simulink model "ur5bh_JustFollow"  (R2021b)
settings: Solver=ode23  StartTime=0.0  StopTime=13  FixedStep=1e-4  MaxStep=1e-3  RelTol=1e-2  AbsTol=1e-2
values from neighbouring files (symbols this model uses):
  Act_Hand = zeros(Phase_Num,1)    [Event2Action.m]
  Act_Lift = zeros(Phase_Num,1)    [Event2Action.m]
  Act_Planner = zeros(Phase_Num,1)    [Event2Action.m]
  Act_Time = zeros(Phase_Num,1)    [Event2Action.m]
  Act_XYZ = zeros(Phase_Num,3)    [Event2Action.m]
  Act_YPR = zeros(Phase_Num,3)    [Event2Action.m]
  maxIter = 200    [Fri_Lancher.m]    (also in ur5bhLancher.m)
undefined symbols (not defined in the file or in its folder): X, Y, Z
libraries: sm_lib x186, nesl_utility x38, robotmaniplib x2, simulink x1
(part 1 of 5)
settings Model: Creator=jobs  LastModifiedBy=jobs

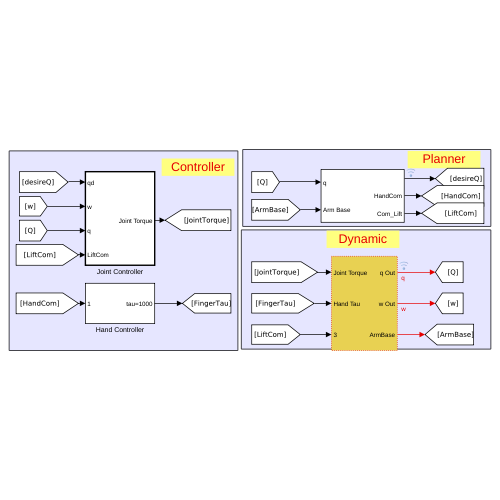
[thumbnail: Simulink's stored preview of the top-level diagram]
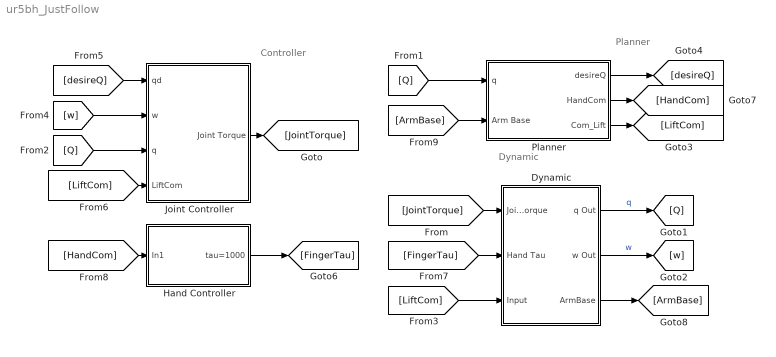
== system ur5bh_JustFollow ==
  note: Dynamic
  note: Planner
  note: Controller
  Dynamic : Subsystem
      settings: MinAlgLoopOccurrences=on
  Hand Controller : Subsystem
  Joint Controller : Subsystem  TreatAsAtomicUnit=on  SystemSampleTime=1e-3
  Planner : Subsystem
  wires:
  Joint Controller/1(Joint Torque) -> [JointTorque]
  [JointTorque] -> Dynamic/1(Joint Torque)
  [Q] -> Planner/1(q)
  [Q] -> Joint Controller/3(q)
  Dynamic/1(q Out) -> [Q]  "q"
  [w] -> Joint Controller/2(w)
  Dynamic/2(w Out) -> [w]  "w"
  Planner/1(desireQ) -> [desireQ]
  [desireQ] -> Joint Controller/1(qd)
  [FingerTau] -> Dynamic/2(Hand Tau)
  Planner/2(HandCom) -> [HandCom]
  [HandCom] -> Hand Controller/1(In1)
  Hand Controller/1(tau=1000) -> [FingerTau]
  Dynamic/3(ArmBase) -> [ArmBase]
  [ArmBase] -> Planner/2(Arm Base)
  [LiftCom] -> Dynamic/3(Input)
  Planner/3(Com_Lift) -> [LiftCom]
  [LiftCom] -> Joint Controller/4(LiftCom)

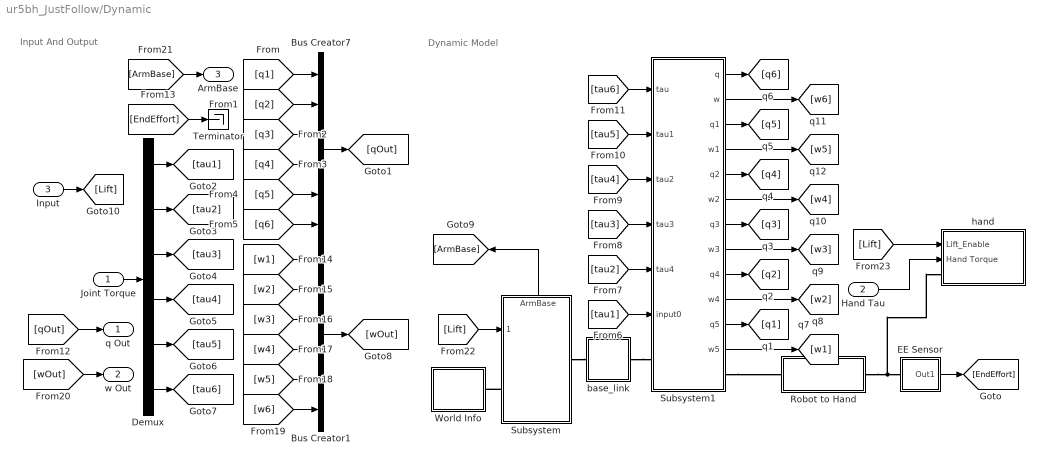
== system ur5bh_JustFollow/Dynamic ==
  note: Dynamic Model
  note: Input And Output
  Joint Torque : Inport
  Hand Tau : Inport  Port=2
  Input : Inport  Port=3
  Bus Creator1 : BusCreator  Inputs=6
  Bus Creator7 : BusCreator  Inputs=6
  Demux : Demux  Outputs=6
  EE Sensor : Subsystem
      settings: PortSchema="{\"entries\":[{\"content\":{\"sides\":[{\"content\":{\"connectorIds\":[\"Out1\"]},\"type\":\"ConnectorPlacement.EquallySpacedRectSide\",\"uuid\":\"1821bd9e-34df-46f7-8d9b-73402f01dbc0\"},{\"content\":{\"connectorIds\":[\"RConn1\"],\"side\":\"RIGHT\"},\"type\":\"ConnectorPlacement.EquallySpacedRectSide\",\"uuid\":\"cfe01d0d-0504-46d0-96c4-84d5e751aaf1\"},{\"content\":{\"connectorIds\":[],\"side\":\"TOP\"},\"type\":\"ConnectorPlacement.EquallySpacedRectSide\",\"uuid\":\"fb6ec0bf-6e00-4c48-b353-ee97f79f22fa\"},{\"content\":{\"connectorIds\":[],\"side\":\"BOTTOM\"},\"type\":\"ConnectorPlacement.EquallySpacedRectSide\",\"uuid\":\"6688a5de-4d5c-429f-9ca8-418d1bff595a\"}]},\"type\":\"ConnectorPlacement.EquallySpacedConnector\",\"uuid\":\"28678e19-8d3c-4397-9fe9-d3bc3a97349c\"}],\"packageUris\":[\"http://schema.mathworks.com/mf0/Connector/R2020b\"],\"version\":\"1.0\"}"
  Robot to Hand : Subsystem
  Subsystem : Subsystem
      settings: PortSchema="{\"entries\":[{\"content\":{\"sides\":[{\"content\":{\"connectorIds\":[\"In1\",\"LConn1\"]},\"type\":\"ConnectorPlacement.EquallySpacedRectSide\",\"uuid\":\"bc59e900-8a65-4f97-be81-06510ea807f2\"},{\"content\":{\"connectorIds\":[\"RConn1\"],\"side\":\"RIGHT\"},\"type\":\"ConnectorPlacement.EquallySpacedRectSide\",\"uuid\":\"d313dc58-bf09-4757-872f-ead6b7b748b5\"},{\"content\":{\"connectorIds\":[\"Out1\"],\"side\":\"TOP\"},\"type\":\"ConnectorPlacement.EquallySpacedRectSide\",\"uuid\":\"71a2b965-5ff9-406f-a52d-ddc68be5512a\"}]},\"type\":\"ConnectorPlacement.EquallySpacedConnector\",\"uuid\":\"b8c6ee35-7b15-4dbb-9c01-21bfdc5f9d27\"}],\"packageUris\":[\"http://schema.mathworks.com/mf0/Connector/R2020b\"],\"version\":\"1.0\"}"
  Subsystem1 : Subsystem
  Terminator : Terminator
  World Info : Subsystem
  base_link : Subsystem
  hand : Subsystem
      settings: PortSchema="{\"entries\":[{\"content\":{\"sides\":[{\"content\":{\"connectorIds\":[\"LConn1\",\"In1\",\"In2\"]},\"type\":\"ConnectorPlacement.EquallySpacedRectSide\",\"uuid\":\"f2c357b2-68da-4259-b6da-bbea843ff329\"},{\"content\":{\"connectorIds\":[],\"side\":\"RIGHT\"},\"type\":\"ConnectorPlacement.EquallySpacedRectSide\",\"uuid\":\"f9d07959-d136-4bfc-946e-50d35ee94d24\"},{\"content\":{\"connectorIds\":[],\"side\":\"TOP\"},\"type\":\"ConnectorPlacement.EquallySpacedRectSide\",\"uuid\":\"c38706b4-1127-4432-a529-c8f32df5cedd\"}]},\"type\":\"ConnectorPlacement.EquallySpacedConnector\",\"uuid\":\"2d678840-68fd-4e92-9d1f-adc30b555a47\"}],\"packageUris\":[\"http://schema.mathworks.com/mf0/Connector/R2020b\"],\"version\":\"1.0\"}"
  q Out : Outport
  w Out : Outport  Port=2
  ArmBase : Outport  Port=3
  wires:
  Demux/6 -> [tau6]
  [q1] -> Bus Creator7/1
  [q3] -> Bus Creator7/3
  Joint Torque/1 -> Demux/1
  Demux/4 -> [tau4]
  [q2] -> Bus Creator7/2
  [q5] -> Bus Creator7/5
  Bus Creator7/1 -> [qOut]
  Demux/3 -> [tau3]
  [qOut] -> q Out/1
  [q6] -> Bus Creator7/6
  [q4] -> Bus Creator7/4
  Demux/2 -> [tau2]
  Demux/1 -> [tau1]
  Demux/5 -> [tau5]
  [w2] -> Bus Creator1/2
  [w3] -> Bus Creator1/3
  [w5] -> Bus Creator1/5
  Bus Creator1/1 -> [wOut]
  [w4] -> Bus Creator1/4
  [w6] -> Bus Creator1/6
  [w1] -> Bus Creator1/1
  [wOut] -> w Out/1
  EE Sensor/1(Out1) -> [EndEffort]
  Hand Tau/1 -> hand/1(Hand Torque)
  [ArmBase] -> ArmBase/1
  [tau6] -> Subsystem1/1(tau)
  [tau5] -> Subsystem1/2(tau1)
  [tau4] -> Subsystem1/3(tau2)
  [tau3] -> Subsystem1/4(tau3)
  [tau2] -> Subsystem1/5(tau4)
  [tau1] -> Subsystem1/6(input0)
  Subsystem1/1(q) -> [q6]
  Subsystem1/2(w) -> [w6]
  Subsystem1/3(q1) -> [q5]
  Subsystem1/4(w1) -> [w5]
  Subsystem1/5(q2) -> [q4]
  Subsystem1/6(w2) -> [w4]
  Subsystem1/7(q3) -> [q3]
  Subsystem1/8(w3) -> [w3]
  Subsystem1/9(q4) -> [q2]
  Subsystem1/10(w4) -> [w2]
  Subsystem1/11(q5) -> [q1]
  Subsystem1/12(w5) -> [w1]
  [EndEffort] -> Terminator/1
  Subsystem/1(ArmBase) -> [ArmBase]
  Input/1 -> [Lift]
  [Lift] -> Subsystem/1(Enable)
  [Lift] -> hand/2(Lift_Enable)
  connections:
  Robot to Hand/RConn1 -- hand/LConn1 -- EE Sensor/RConn1
  base_link/RConn1 -- Subsystem1/LConn1
  Subsystem1/RConn1 -- Robot to Hand/LConn1
  Subsystem/RConn1 -- base_link/LConn1
  Subsystem/LConn1 -- World Info/RConn1

== system ur5bh_JustFollow/Hand Controller ==
  In1 : Inport
  MATLAB Function : MATLAB Function  TreatAsAtomicUnit=on
  tau=1000 : Outport
  wires:
  MATLAB Function/1(y) -> tau=1000/1
  In1/1 -> MATLAB Function/1(u)

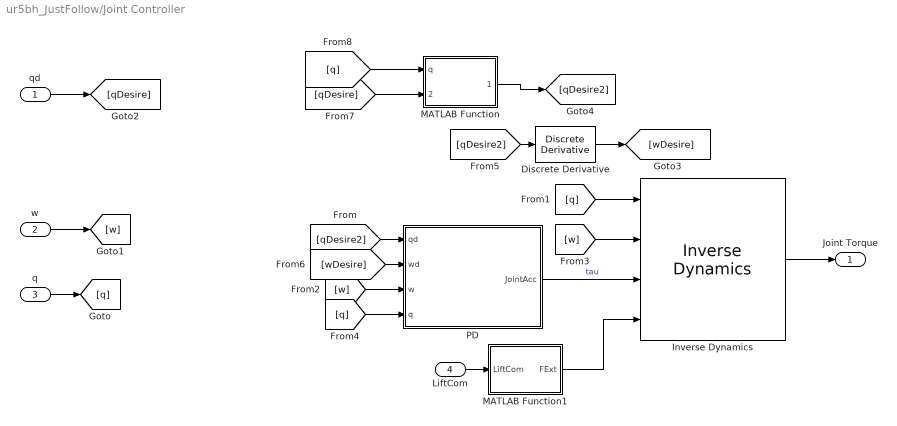
== system ur5bh_JustFollow/Joint Controller ==
  qd : Inport
  w : Inport  Port=2
  q : Inport  Port=3
  LiftCom : Inport  Port=4
  Discrete Derivative : simulink/Discrete/Discrete Derivative  gainval=1.0  ICPrevScaledInput=0.0  OutMin=[]  OutMax=[]  OutDataType=fixdt(1, 16)  OutScaling=2^-10  DoSatur=off
  "Inverse Dynamics " : robotmaniplib/Inverse Dynamics  RigidBodyTree=ur5_InverseDynamic  SimulateUsing=Interpreted execution
      settings: SourceProductBaseCode=RO
  MATLAB Function : MATLAB Function  TreatAsAtomicUnit=on
  MATLAB Function1 : MATLAB Function  TreatAsAtomicUnit=on
  PD : MATLAB Function  TreatAsAtomicUnit=on
  Joint Torque : Outport
  wires:
  "Inverse Dynamics "/1 -> Joint Torque/1
  q/1 -> [q]
  [q] -> "Inverse Dynamics "/1
  w/1 -> [w]
  [w] -> PD/3(w)
  [w] -> "Inverse Dynamics "/2
  [q] -> PD/4(q)
  PD/1(JointAcc) -> "Inverse Dynamics "/3  "tau"
  MATLAB Function1/1(FExt) -> "Inverse Dynamics "/4
  qd/1 -> [qDesire]
  [qDesire2] -> PD/1(qd)
  [qDesire2] -> Discrete Derivative/1
  Discrete Derivative/1 -> [wDesire]
  [wDesire] -> PD/2(wd)
  [qDesire] -> MATLAB Function/2(desireQ)
  MATLAB Function/1(desireQ2) -> [qDesire2]
  [q] -> MATLAB Function/1(q)
  LiftCom/1 -> MATLAB Function1/1(LiftCom)

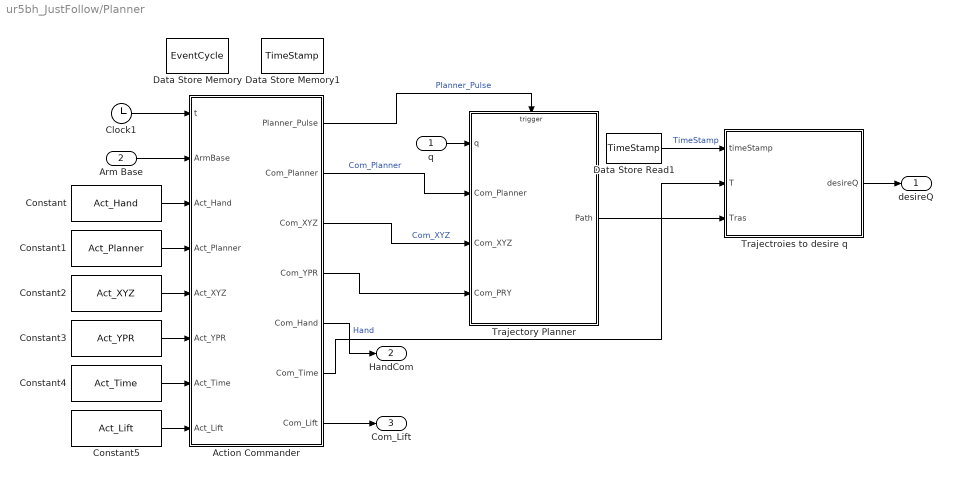
== system ur5bh_JustFollow/Planner ==
  q : Inport
  Arm Base : Inport  Port=2
  Action Commander : MATLAB Function  TreatAsAtomicUnit=on  SystemSampleTime=1e-3
  Clock1 : Clock
  Constant : Constant  Value=Act_Hand
  Constant1 : Constant  Value=Act_Planner
  Constant2 : Constant  Value=Act_XYZ
  Constant3 : Constant  Value=Act_YPR
  Constant4 : Constant  Value=Act_Time
  Constant5 : Constant  Value=Act_Lift
  Data Store Memory : DataStoreMemory  DataStoreName=EventCycle  InitialValue=1  ShareAcrossModelInstances=on  ShowAdditionalParam=off  OutMin=0  OutDataTypeStr=int64  Dimensions=1
  Data Store Memory1 : DataStoreMemory  DataStoreName=TimeStamp  ShareAcrossModelInstances=on  ShowAdditionalParam=off  OutMin=0  OutDataTypeStr=double  Dimensions=1
  Data Store Read1 : DataStoreRead  DataStoreName=TimeStamp  IndexOptions=Index vector (dialog)  Indices=1  OutputSizes=1
  Trajectory Planner : Subsystem  TreatAsAtomicUnit=on
  Trajectroies to desire q : MATLAB Function  TreatAsAtomicUnit=on
  desireQ : Outport
  HandCom : Outport  Port=2
  Com_Lift : Outport  Port=3
  wires:
  Clock1/1 -> Action Commander/1(t)
  Action Commander/1(Planner_Pulse) -> Trajectory Planner/Trigger  "Planner_Pulse"
  Trajectroies to desire q/1(desireQ) -> desireQ/1
  q/1 -> Trajectory Planner/1(q)
  Data Store Read1/1 -> Trajectroies to desire q/1(timeStamp)  "TimeStamp"
  Action Commander/6(Com_Time) -> Trajectroies to desire q/2(T)
  Constant/1 -> Action Commander/3(Act_Hand)
  Action Commander/5(Com_Hand) -> HandCom/1  "Hand"
  Constant2/1 -> Action Commander/5(Act_XYZ)
  Constant3/1 -> Action Commander/6(Act_YPR)
  Constant4/1 -> Action Commander/7(Act_Time)
  Arm Base/1 -> Action Commander/2(ArmBase)
  Constant1/1 -> Action Commander/4(Act_Planner)
  Action Commander/3(Com_XYZ) -> Trajectory Planner/3(Com_XYZ)  "Com_XYZ"
  Action Commander/4(Com_YPR) -> Trajectory Planner/4(Com_PRY)
  Action Commander/2(Com_Planner) -> Trajectory Planner/2(Com_Planner)  "Com_Planner"
  Trajectory Planner/1(Path) -> Trajectroies to desire q/3(Tras)
  Constant5/1 -> Action Commander/8(Act_Lift)
  Action Commander/7(Com_Lift) -> Com_Lift/1

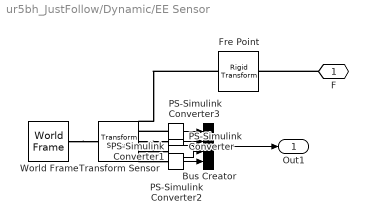
== system ur5bh_JustFollow/Dynamic/EE Sensor ==
  Bus Creator : BusCreator  Inputs=4
  Fre Point : sm_lib/Frames and Transforms/Rigid Transform  TranslationMethod=Cartesian  TranslationStandardOffset=0  TranslationLengthUnit=m  TranslationStandardAxis=+Z  TranslationCartesianOffset=[0, 0, 0.12]  TranslationROffset=0  TranslationROffsetUnits=m  TranslationZOffset=0  TranslationZOffsetUnits=m  TranslationThetaOffset=0  TranslationThetaOffsetUnits=deg  RotationMethod=RotationSequence  RotationAngleUnits=deg  RotationStandardAxis=+Z  RotationAngle=0.0  RotationArbitraryAxis=[0 0 1]  FollAlignAxisA=+X  BaseAlignAxisA=+Y  FollAlignAxisB=+Y  BaseAlignAxisB=+Z  RotationSequenceAxes=BaseAxes  RotationSequence=XYZ  RotationSequenceAngles=[0, 0, 0]  RotationSequenceAnglesUnits=rad  RotationMatrix=[1 0 0; 0 1 0; 0 0 1]
  PS-Simulink Converter{,1..3} (4 alike) : nesl_utility/PS-Simulink Converter  PhysicalDomain=network_engine_domain  SubClassName=ps_output  LeftPortType=input  RightPortType=output  PseudoPeriodic=off  Frequencies=[]  Unit=inherit  AffineConversion=off
      settings: SourceProductBaseCode=PW,SS
  Transform Sensor : sm_lib/Frames and Transforms/Transform Sensor  MeasurementFrame=World  SenseAngle=off  SenseAxis=off  SenseAngle1=off  SenseAngle2=off  SenseAngle3=off  SenseQ=on  SenseR=off  SenseOmegaX=off  SenseOmegaY=off  SenseOmegaZ=off  SenseOmega1=off  SenseOmega2=off  SenseOmega3=off  SenseQDot=off  SenseRDot=off  SenseAlphaX=off  SenseAlphaY=off  SenseAlphaZ=off  SenseAlpha1=off  SenseAlpha2=off  SenseAlpha3=off  SenseQDDot=off  SenseRDDot=off  SenseX=on  SenseY=on  SenseZ=on  SenseRad=off  SenseAzim=off  SenseDist=off  SenseInc=off  SenseXDot=off  SenseYDot=off  SenseZDot=off  SenseRadDot=off  SenseAzimDot=off  SenseDistDot=off  SenseIncDot=off  SenseXDDot=off  SenseYDDot=off  SenseZDDot=off  SenseRadDDot=off  SenseAzimDDot=off  SenseDistDDot=off  SenseIncDDot=off
  World Frame : sm_lib/Frames and Transforms/World Frame
  F : PMIOPort  Side=Right
  Out1 : Outport
  wires:
  Bus Creator/1 -> Out1/1
  PS-Simulink Converter3/1 -> Bus Creator/1
  PS-Simulink Converter1/1 -> Bus Creator/3
  PS-Simulink Converter/1 -> Bus Creator/2
  PS-Simulink Converter2/1 -> Bus Creator/4
  connections:
  PS-Simulink Converter3/LConn1 -- Transform Sensor/RConn2
  Transform Sensor/RConn5 -- PS-Simulink Converter2/LConn1
  Transform Sensor/RConn4 -- PS-Simulink Converter1/LConn1
  Transform Sensor/RConn3 -- PS-Simulink Converter/LConn1
  World Frame/RConn1 -- Transform Sensor/LConn1
  F/RConn1 -- Fre Point/LConn1
  Fre Point/RConn1 -- Transform Sensor/RConn1

== system ur5bh_JustFollow/Dynamic/Robot to Hand ==
  bh_base_joint : sm_lib/Joints/Weld Joint  JointMode=Normal  SenseConstraintForce=off  SenseConstraintForceX=off  SenseConstraintForceY=off  SenseConstraintForceZ=off  SenseConstraintTorque=off  SenseConstraintTorqueX=off  SenseConstraintTorqueY=off  SenseConstraintTorqueZ=off  SenseTotalForce=off  SenseTotalForceX=off  SenseTotalForceY=off  SenseTotalForceZ=off  SenseTotalTorque=off  SenseTotalTorqueX=off  SenseTotalTorqueY=off  SenseTotalTorqueZ=off  CompositeWrenchDir=FollowerOnBase  CompositeWrenchFrame=BaseFrame
  ur5 End Effort : Subsystem
  Conn1 : PMIOPort  Side=Right
  Conn2 : PMIOPort  Port=2  Side=Left
  connections:
  ur5 End Effort/RConn1 -- bh_base_joint/LConn1
  Conn2/RConn1 -- ur5 End Effort/LConn1
  bh_base_joint/RConn1 -- Conn1/RConn1

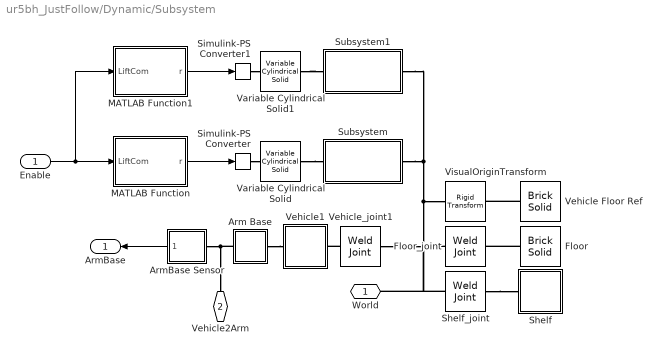
== system ur5bh_JustFollow/Dynamic/Subsystem ==
  Enable : Inport
  Arm Base : Subsystem
  ArmBase Sensor : Subsystem
      settings: PortSchema="{\"entries\":[{\"content\":{\"sides\":[{\"content\":{\"connectorIds\":[\"Out1\"]},\"type\":\"ConnectorPlacement.EquallySpacedRectSide\",\"uuid\":\"1821bd9e-34df-46f7-8d9b-73402f01dbc0\"},{\"content\":{\"connectorIds\":[\"RConn1\"],\"side\":\"RIGHT\"},\"type\":\"ConnectorPlacement.EquallySpacedRectSide\",\"uuid\":\"cfe01d0d-0504-46d0-96c4-84d5e751aaf1\"},{\"content\":{\"connectorIds\":[],\"side\":\"TOP\"},\"type\":\"ConnectorPlacement.EquallySpacedRectSide\",\"uuid\":\"fb6ec0bf-6e00-4c48-b353-ee97f79f22fa\"}]},\"type\":\"ConnectorPlacement.EquallySpacedConnector\",\"uuid\":\"28678e19-8d3c-4397-9fe9-d3bc3a97349c\"}],\"packageUris\":[\"http://schema.mathworks.com/mf0/Connector/R2020b\"],\"version\":\"1.0\"}"
  Floor : sm_lib/Body Elements/Brick Solid  GraphicAmbientColor=[0.15 0.15 0.15 1.0]  BasedOnType=Density  BrickDimensions=[3 3 0.0001]  BrickDimensionUnits=m  CenterOfMass=[0 0 0]  CenterOfMassUnits=m  GraphicDiffuseColor=[0.5 0.5 0.5]  Density=1000  DensityUnits=kg/m^3  DoExposeReferenceFrame=on  GraphicEmissiveColor=[0.0 0.0 0.0 1.0]  ExportEntireGeometry=off  SerializedFrames=<Frames/>  MarkerShape=Sphere  MarkerSize=10  GraphicType=FromGeometry  InertiaType=CalculateFromGeometry  Mass=1  MassUnits=kg  MomentsOfInertia=[1 1 1]  MomentsOfInertiaUnits=kg*m^2  GraphicOpacity=1.0  ProductsOfInertia=[0 0 0]  ProductsOfInertiaUnits=kg*m^2  GraphicShininess=75  GraphicSpecularColor=[0.5 0.5 0.5 1.0]  GraphicVisPropType=SimpleVisualProperties
  Floor_joint : sm_lib/Joints/Weld Joint  JointMode=Normal  SenseConstraintForce=off  SenseConstraintForceX=off  SenseConstraintForceY=off  SenseConstraintForceZ=off  SenseConstraintTorque=off  SenseConstraintTorqueX=off  SenseConstraintTorqueY=off  SenseConstraintTorqueZ=off  SenseTotalForce=off  SenseTotalForceX=off  SenseTotalForceY=off  SenseTotalForceZ=off  SenseTotalTorque=off  SenseTotalTorqueX=off  SenseTotalTorqueY=off  SenseTotalTorqueZ=off  CompositeWrenchDir=FollowerOnBase  CompositeWrenchFrame=BaseFrame
  MATLAB Function : MATLAB Function  TreatAsAtomicUnit=on
  MATLAB Function1 : MATLAB Function  TreatAsAtomicUnit=on
  Shelf : Subsystem
  Shelf_joint : sm_lib/Joints/Weld Joint  JointMode=Normal  SenseConstraintForce=off  SenseConstraintForceX=off  SenseConstraintForceY=off  SenseConstraintForceZ=off  SenseConstraintTorque=off  SenseConstraintTorqueX=off  SenseConstraintTorqueY=off  SenseConstraintTorqueZ=off  SenseTotalForce=off  SenseTotalForceX=off  SenseTotalForceY=off  SenseTotalForceZ=off  SenseTotalTorque=off  SenseTotalTorqueX=off  SenseTotalTorqueY=off  SenseTotalTorqueZ=off  CompositeWrenchDir=FollowerOnBase  CompositeWrenchFrame=BaseFrame
  Simulink-PS Converter : nesl_utility/Simulink-PS Converter  PhysicalDomain=network_engine_domain  SubClassName=ps_input  LeftPortType=input  RightPortType=output  PseudoPeriodic=off  Frequencies=[]  NoiseDistribution=none  NoiseParameters=[]  Unit=1  AffineConversion=off  FilteringAndDerivatives=provide  SimscapeFilterOrder=1  InputFilterTimeConstant=0.001  UdotUserProvided=0
      settings: SourceProductBaseCode=PW,SS
  Simulink-PS Converter1 : nesl_utility/Simulink-PS Converter  PhysicalDomain=network_engine_domain  SubClassName=ps_input  LeftPortType=input  RightPortType=output  PseudoPeriodic=off  Frequencies=[]  NoiseDistribution=none  NoiseParameters=[]  Unit=1  AffineConversion=off  FilteringAndDerivatives=provide  SimscapeFilterOrder=1  InputFilterTimeConstant=0.001  UdotUserProvided=0
      settings: SourceProductBaseCode=PW,SS
  Subsystem : Subsystem
  Subsystem1 : Subsystem
  Variable Cylindrical Solid : sm_lib/Body Elements/Variable Mass/Variable Cylindrical Solid  LengthType=Constant  Length=0.12  LengthUnits=m  RadiusType=ProvidedByInput  Radius=1  RadiusUnits=m  MassType=CalculateFromGeometry  InitialMassType=Specified  InitialMass=1  InitialMassUnits=kg  Density=1  DensityUnits=kg/m^3  SenseRadius=off  SenseLength=off  SenseMass=off  SenseCenterOfMass=off  SenseInertiaMatrix=off  GraphicType=FromGeometry  MarkerShape=Sphere  MarkerSize=10  GraphicVisPropType=SimpleVisualProperties  GraphicDiffuseColor=[0.5 0.5 0.5]  GraphicSpecularColor=[0.5 0.5 0.5 1.0]  GraphicAmbientColor=[0.15 0.15 0.15 1.0]  GraphicEmissiveColor=[0.0 0.0 0.0 1.0]  GraphicShininess=75  GraphicOpacity=1.0
      settings: SourceProductBaseCode=MS
  Variable Cylindrical Solid1 : sm_lib/Body Elements/Variable Mass/Variable Cylindrical Solid  LengthType=Constant  Length=0.12  LengthUnits=m  RadiusType=ProvidedByInput  Radius=1  RadiusUnits=m  MassType=CalculateFromGeometry  InitialMassType=Specified  InitialMass=1  InitialMassUnits=kg  Density=1  DensityUnits=kg/m^3  SenseRadius=off  SenseLength=off  SenseMass=off  SenseCenterOfMass=off  SenseInertiaMatrix=off  GraphicType=FromGeometry  MarkerShape=Sphere  MarkerSize=10  GraphicVisPropType=SimpleVisualProperties  GraphicDiffuseColor=[0.5 0.5 0.5]  GraphicSpecularColor=[0.5 0.5 0.5 1.0]  GraphicAmbientColor=[0.15 0.15 0.15 1.0]  GraphicEmissiveColor=[0.0 0.0 0.0 1.0]  GraphicShininess=75  GraphicOpacity=1.0
      settings: SourceProductBaseCode=MS
  Vehicle Floor Ref : sm_lib/Body Elements/Brick Solid  GraphicAmbientColor=[0.15 0.15 0.15 1.0]  BasedOnType=Density  BrickDimensions=[1.5 0.8 0.01]  BrickDimensionUnits=m  CenterOfMass=[0 0 0]  CenterOfMassUnits=m  GraphicDiffuseColor=[1.0 0.0 0.0]  Density=1000  DensityUnits=kg/m^3  DoExposeReferenceFrame=on  GraphicEmissiveColor=[0.0 0.0 0.0 1.0]  ExportEntireGeometry=off  SerializedFrames=<Frames/>  MarkerShape=Sphere  MarkerSize=10  GraphicType=FromGeometry  InertiaType=CalculateFromGeometry  Mass=1  MassUnits=kg  MomentsOfInertia=[1 1 1]  MomentsOfInertiaUnits=kg*m^2  GraphicOpacity=1.0  ProductsOfInertia=[0 0 0]  ProductsOfInertiaUnits=kg*m^2  GraphicShininess=75  GraphicSpecularColor=[0.5 0.5 0.5 1.0]  GraphicVisPropType=SimpleVisualProperties
  Vehicle1 : Subsystem
  Vehicle_joint1 : sm_lib/Joints/Weld Joint  JointMode=Normal  SenseConstraintForce=off  SenseConstraintForceX=off  SenseConstraintForceY=off  SenseConstraintForceZ=off  SenseConstraintTorque=off  SenseConstraintTorqueX=off  SenseConstraintTorqueY=off  SenseConstraintTorqueZ=off  SenseTotalForce=off  SenseTotalForceX=off  SenseTotalForceY=off  SenseTotalForceZ=off  SenseTotalTorque=off  SenseTotalTorqueX=off  SenseTotalTorqueY=off  SenseTotalTorqueZ=off  CompositeWrenchDir=FollowerOnBase  CompositeWrenchFrame=BaseFrame
  VisualOriginTransform : sm_lib/Frames and Transforms/Rigid Transform  TranslationMethod=Cartesian  TranslationStandardOffset=0  TranslationLengthUnit=m  TranslationStandardAxis=+Z  TranslationCartesianOffset=[0.75, 0, 0.28]  TranslationROffset=0  TranslationROffsetUnits=m  TranslationZOffset=0  TranslationZOffsetUnits=m  TranslationThetaOffset=0  TranslationThetaOffsetUnits=deg  RotationMethod=None  RotationAngleUnits=rad  RotationStandardAxis=+Z  RotationAngle=pi/2  RotationArbitraryAxis=[1 0 0]  FollAlignAxisA=+X  BaseAlignAxisA=+Y  FollAlignAxisB=+Y  BaseAlignAxisB=+Z  RotationSequenceAxes=BaseAxes  RotationSequence=XYZ  RotationSequenceAngles=0  RotationSequenceAnglesUnits=rad  RotationMatrix=[1 0 0; 0 1 0; 0 0 1]
  World : PMIOPort  Side=Left
  Vehicle2Arm : PMIOPort  Port=2  Side=Right
  ArmBase : Outport
  wires:
  ArmBase Sensor/1(Out1) -> ArmBase/1
  MATLAB Function/1(r) -> Simulink-PS Converter/1
  Enable/1 -> MATLAB Function1/1(LiftCom), MATLAB Function/1(LiftCom)
  MATLAB Function1/1(r) -> Simulink-PS Converter1/1
  connections:
  Subsystem/LConn1 -- VisualOriginTransform/LConn1 -- Floor_joint/LConn1 -- Vehicle_joint1/LConn1 -- World/RConn1 -- Shelf_joint/LConn1 -- Subsystem1/LConn1
  ArmBase Sensor/RConn1 -- Arm Base/RConn1 -- Vehicle2Arm/RConn1
  Variable Cylindrical Solid/RConn1 -- Subsystem/RConn1
  Simulink-PS Converter/RConn1 -- Variable Cylindrical Solid/LConn1
  Shelf_joint/RConn1 -- Shelf/LConn1
  Vehicle_joint1/RConn1 -- Vehicle1/LConn1
  Arm Base/LConn1 -- Vehicle1/RConn1
  Floor/RConn1 -- Floor_joint/RConn1
  Vehicle Floor Ref/RConn1 -- VisualOriginTransform/RConn1
  Variable Cylindrical Solid1/RConn1 -- Subsystem1/RConn1
  Simulink-PS Converter1/RConn1 -- Variable Cylindrical Solid1/LConn1

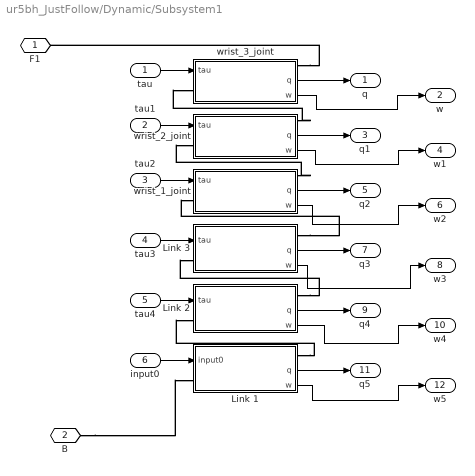
== system ur5bh_JustFollow/Dynamic/Subsystem1 ==
  tau : Inport
  tau1 : Inport  Port=2
  tau2 : Inport  Port=3
  tau3 : Inport  Port=4
  tau4 : Inport  Port=5
  input0 : Inport  Port=6
  Link 1 : Subsystem
      settings: PortSchema="{\"entries\":[{\"content\":{\"sides\":[{\"content\":{\"connectorIds\":[\"In1\",\"LConn1\"]},\"type\":\"ConnectorPlacement.EquallySpacedRectSide\",\"uuid\":\"41f6cf96-6caa-4c29-b424-a0af70ff3cad\"},{\"content\":{\"connectorIds\":[\"RConn1\",\"Out1\",\"Out2\"],\"side\":\"RIGHT\"},\"type\":\"ConnectorPlacement.EquallySpacedRectSide\",\"uuid\":\"f3077720-0bbe-4c8a-929f-ab241397ae87\"},{\"content\":{\"connectorIds\":[],\"side\":\"TOP\"},\"type\":\"ConnectorPlacement.EquallySpacedRectSide\",\"uuid\":\"968fa520-708e-401a-afd3-f1d2650f98d2\"}]},\"type\":\"ConnectorPlacement.EquallySpacedConnector\",\"uuid\":\"bca11362-a401-4867-9a4d-3d2cb5381415\"}],\"packageUris\":[\"http://schema.mathworks.com/mf0/Connector/R2020b\"],\"version\":\"1.0\"}"
  Link 2 : Subsystem
      settings: PortSchema="{\"entries\":[{\"content\":{\"sides\":[{\"content\":{\"connectorIds\":[\"In1\",\"LConn1\"]},\"type\":\"ConnectorPlacement.EquallySpacedRectSide\",\"uuid\":\"41f6cf96-6caa-4c29-b424-a0af70ff3cad\"},{\"content\":{\"connectorIds\":[\"RConn1\",\"Out1\",\"Out2\"],\"side\":\"RIGHT\"},\"type\":\"ConnectorPlacement.EquallySpacedRectSide\",\"uuid\":\"f3077720-0bbe-4c8a-929f-ab241397ae87\"},{\"content\":{\"connectorIds\":[],\"side\":\"TOP\"},\"type\":\"ConnectorPlacement.EquallySpacedRectSide\",\"uuid\":\"968fa520-708e-401a-afd3-f1d2650f98d2\"}]},\"type\":\"ConnectorPlacement.EquallySpacedConnector\",\"uuid\":\"bca11362-a401-4867-9a4d-3d2cb5381415\"}],\"packageUris\":[\"http://schema.mathworks.com/mf0/Connector/R2020b\"],\"version\":\"1.0\"}"
  Link 3 : Subsystem
      settings: PortSchema="{\"entries\":[{\"content\":{\"sides\":[{\"content\":{\"connectorIds\":[\"In1\",\"LConn1\"]},\"type\":\"ConnectorPlacement.EquallySpacedRectSide\",\"uuid\":\"41f6cf96-6caa-4c29-b424-a0af70ff3cad\"},{\"content\":{\"connectorIds\":[\"RConn1\",\"Out1\",\"Out2\"],\"side\":\"RIGHT\"},\"type\":\"ConnectorPlacement.EquallySpacedRectSide\",\"uuid\":\"f3077720-0bbe-4c8a-929f-ab241397ae87\"},{\"content\":{\"connectorIds\":[],\"side\":\"TOP\"},\"type\":\"ConnectorPlacement.EquallySpacedRectSide\",\"uuid\":\"968fa520-708e-401a-afd3-f1d2650f98d2\"}]},\"type\":\"ConnectorPlacement.EquallySpacedConnector\",\"uuid\":\"bca11362-a401-4867-9a4d-3d2cb5381415\"}],\"packageUris\":[\"http://schema.mathworks.com/mf0/Connector/R2020b\"],\"version\":\"1.0\"}"
  wrist_1_joint : Subsystem
      settings: PortSchema="{\"entries\":[{\"content\":{\"sides\":[{\"content\":{\"connectorIds\":[\"In1\",\"LConn1\"]},\"type\":\"ConnectorPlacement.EquallySpacedRectSide\",\"uuid\":\"41f6cf96-6caa-4c29-b424-a0af70ff3cad\"},{\"content\":{\"connectorIds\":[\"RConn1\",\"Out1\",\"Out2\"],\"side\":\"RIGHT\"},\"type\":\"ConnectorPlacement.EquallySpacedRectSide\",\"uuid\":\"f3077720-0bbe-4c8a-929f-ab241397ae87\"},{\"content\":{\"connectorIds\":[],\"side\":\"TOP\"},\"type\":\"ConnectorPlacement.EquallySpacedRectSide\",\"uuid\":\"968fa520-708e-401a-afd3-f1d2650f98d2\"}]},\"type\":\"ConnectorPlacement.EquallySpacedConnector\",\"uuid\":\"bca11362-a401-4867-9a4d-3d2cb5381415\"}],\"packageUris\":[\"http://schema.mathworks.com/mf0/Connector/R2020b\"],\"version\":\"1.0\"}"
  wrist_2_joint : Subsystem
      settings: PortSchema="{\"entries\":[{\"content\":{\"sides\":[{\"content\":{\"connectorIds\":[\"In1\",\"LConn1\"]},\"type\":\"ConnectorPlacement.EquallySpacedRectSide\",\"uuid\":\"41f6cf96-6caa-4c29-b424-a0af70ff3cad\"},{\"content\":{\"connectorIds\":[\"RConn1\",\"Out1\",\"Out2\"],\"side\":\"RIGHT\"},\"type\":\"ConnectorPlacement.EquallySpacedRectSide\",\"uuid\":\"f3077720-0bbe-4c8a-929f-ab241397ae87\"},{\"content\":{\"connectorIds\":[],\"side\":\"TOP\"},\"type\":\"ConnectorPlacement.EquallySpacedRectSide\",\"uuid\":\"968fa520-708e-401a-afd3-f1d2650f98d2\"}]},\"type\":\"ConnectorPlacement.EquallySpacedConnector\",\"uuid\":\"bca11362-a401-4867-9a4d-3d2cb5381415\"}],\"packageUris\":[\"http://schema.mathworks.com/mf0/Connector/R2020b\"],\"version\":\"1.0\"}"
  wrist_3_joint : Subsystem
      settings: PortSchema="{\"entries\":[{\"content\":{\"sides\":[{\"content\":{\"connectorIds\":[\"In1\",\"LConn1\"]},\"type\":\"ConnectorPlacement.EquallySpacedRectSide\",\"uuid\":\"41f6cf96-6caa-4c29-b424-a0af70ff3cad\"},{\"content\":{\"connectorIds\":[\"RConn1\",\"Out1\",\"Out2\"],\"side\":\"RIGHT\"},\"type\":\"ConnectorPlacement.EquallySpacedRectSide\",\"uuid\":\"f3077720-0bbe-4c8a-929f-ab241397ae87\"},{\"content\":{\"connectorIds\":[],\"side\":\"TOP\"},\"type\":\"ConnectorPlacement.EquallySpacedRectSide\",\"uuid\":\"968fa520-708e-401a-afd3-f1d2650f98d2\"}]},\"type\":\"ConnectorPlacement.EquallySpacedConnector\",\"uuid\":\"bca11362-a401-4867-9a4d-3d2cb5381415\"}],\"packageUris\":[\"http://schema.mathworks.com/mf0/Connector/R2020b\"],\"version\":\"1.0\"}"
  F1 : PMIOPort  Side=Right
  B : PMIOPort  Port=2  Side=Left
  q : Outport
  w : Outport  Port=2
  q1 : Outport  Port=3
  w1 : Outport  Port=4
  q2 : Outport  Port=5
  w2 : Outport  Port=6
  q3 : Outport  Port=7
  w3 : Outport  Port=8
  q4 : Outport  Port=9
  w4 : Outport  Port=10
  q5 : Outport  Port=11
  w5 : Outport  Port=12
  wires:
  wrist_1_joint/1(q) -> q2/1
  tau3/1 -> Link 3/1(tau)
  wrist_2_joint/1(q) -> q1/1
  wrist_3_joint/2(w) -> w/1
  tau2/1 -> wrist_1_joint/1(tau)
  tau4/1 -> Link 2/1(tau)
  wrist_2_joint/2(w) -> w1/1
  wrist_1_joint/2(w) -> w2/1
  Link 1/2(w) -> w5/1
  tau/1 -> wrist_3_joint/1(tau)
  wrist_3_joint/1(q) -> q/1
  Link 1/1(q) -> q5/1
  Link 2/2(w) -> w4/1
  input0/1 -> Link 1/1(input0)
  Link 3/2(w) -> w3/1
  tau1/1 -> wrist_2_joint/1(tau)
  Link 3/1(q) -> q3/1
  Link 2/1(q) -> q4/1
  connections:
  Link 3/RConn1 -- wrist_1_joint/LConn1
  wrist_2_joint/RConn1 -- wrist_3_joint/LConn1
  wrist_3_joint/RConn1 -- F1/RConn1
  B/RConn1 -- Link 1/LConn1
  wrist_1_joint/RConn1 -- wrist_2_joint/LConn1
  Link 1/RConn1 -- Link 2/LConn1
  Link 2/RConn1 -- Link 3/LConn1

== system ur5bh_JustFollow/Dynamic/World Info ==
  MechanismConfiguration : sm_lib/Utilities/Mechanism Configuration  UniformGravity=Constant  GravityVector=[0 0 -9.80665]  GravityUnits=m/s^2  LinearizationDelta=0.001  JointModeTransitionNonlinearIterations=2
  Solver Configuration : nesl_utility/Solver Configuration  PhysicalDomain=network_engine_domain  SubClassName=solver  LeftPortType=input  RightPortType=generic  Tones=[]  Harmonics=[]  SimulateNoise=off  Profile=off  UseLocalSampling=off  EnableSwitchedLinearOptims=on  FrequencyDomain=off  UseCCode=off  RelTol=0.001  AbsTol=1e-06  MinStep=1e-09  ToWorkspace=off  RevertToSquareIcSolve=off  NumHomotopyIterations=100  PhasorMode=off  PhasorModeNumHarmonics=1  DoDC=off  ResidualTolerance=1e-09  UseLocalSolver=off  LocalSolverChoice=NE_BACKWARD_EULER_ADVANCER  LocalSolverSampleTime=0.001  DoFixedCost=off  MaxNonlinIter=3  MaxModeIter=2  ComputeImpulses=off  ImpulseIterations=2  LinearAlgebra=auto  EquationFormulation=NE_TIME_EF  DelaysMemoryBudget=1024  AutomaticFiltering=on  FilteringTimeConstant=0.001  PartitionStorageMethod=AS_NEEDED  PartitionMemoryBudget=1024  PartitionMethod=ROBUST
      settings: SourceProductBaseCode=PW,SS
  World : sm_lib/Frames and Transforms/World Frame
  Conn1 : PMIOPort  Side=Right
  connections:
  Solver Configuration/RConn1 -- Conn1/RConn1 -- World/RConn1 -- MechanismConfiguration/RConn1

== system ur5bh_JustFollow/Dynamic/base_link ==
  Inertia : sm_lib/Body Elements/Inertia  InertiaType=Custom  Mass=4  MassUnits=kg  CenterOfMass=[0, 0, 0]  CenterOfMassUnits=m  MomentsOfInertia=[0.00443333156, 0.00443333156, 0.0072]  MomentsOfInertiaUnits=kg*m^2  ProductsOfInertia=[0, 0, 0]  ProductsOfInertiaUnits=kg*m^2  GraphicType=None  MarkerShape=Inertia  MarkerSize=20  GraphicVisPropType=SimpleVisualProperties  GraphicDiffuseColor=[0.5 0.5 0.5]  GraphicSpecularColor=[0.5 0.5 0.5 1.0]  GraphicAmbientColor=[0.15 0.15 0.15 1.0]  GraphicEmissiveColor=[0.0 0.0 0.0 1.0]  GraphicShininess=75  GraphicOpacity=1.0
  InertiaOriginTransform : sm_lib/Frames and Transforms/Rigid Transform  TranslationMethod=Cartesian  TranslationStandardOffset=0  TranslationLengthUnit=m  TranslationStandardAxis=+Z  TranslationCartesianOffset=[0, 0, 0]  TranslationROffset=0  TranslationROffsetUnits=m  TranslationZOffset=0  TranslationZOffsetUnits=m  TranslationThetaOffset=0  TranslationThetaOffsetUnits=deg  RotationMethod=RotationSequence  RotationAngleUnits=deg  RotationStandardAxis=+Z  RotationAngle=0.0  RotationArbitraryAxis=[0 0 1]  FollAlignAxisA=+X  BaseAlignAxisA=+Y  FollAlignAxisB=+Y  BaseAlignAxisB=+Z  RotationSequenceAxes=BaseAxes  RotationSequence=XYZ  RotationSequenceAngles=[0, 0, 0]  RotationSequenceAnglesUnits=rad  RotationMatrix=[1 0 0; 0 1 0; 0 0 1]
  ReferenceFrame : sm_lib/Frames and Transforms/Reference Frame
  Visual : sm_lib/Body Elements/File Solid  ExtGeomFileName=ur_description/meshes/ur5/visual/base.stl  UnitType=Custom  ExtGeomFileUnits=m  StepReaderType=HEX  ExportConvexHullGeometry=off  InertiaType=Custom  Mass=0  MassUnits=kg  CenterOfMass=[0, 0, 0]  CenterOfMassUnits=m  MomentsOfInertia=[0, 0, 0]  MomentsOfInertiaUnits=kg*m^2  ProductsOfInertia=[0, 0, 0]  ProductsOfInertiaUnits=kg*m^2  BasedOnType=DensityFromFile  Density=1000  DensityUnits=kg/m^3  DoExposeReferenceFrame=on  SerializedFrames=<Frames/>  GraphicType=FromGeometry  MarkerShape=Sphere  MarkerSize=10  GraphicVisPropType=SimpleVisualProperties  GraphicDiffuseColor=[0.5, 0.5, 0.5]  GraphicSpecularColor=[0.5 0.5 0.5 1.0]  GraphicAmbientColor=[0.15 0.15 0.15 1.0]  GraphicEmissiveColor=[0.0 0.0 0.0 1.0]  GraphicShininess=75  GraphicOpacity=1
  VisualOriginTransform : sm_lib/Frames and Transforms/Rigid Transform  TranslationMethod=Cartesian  TranslationStandardOffset=0  TranslationLengthUnit=m  TranslationStandardAxis=+Z  TranslationCartesianOffset=[0, 0, 0]  TranslationROffset=0  TranslationROffsetUnits=m  TranslationZOffset=0  TranslationZOffsetUnits=m  TranslationThetaOffset=0  TranslationThetaOffsetUnits=deg  RotationMethod=RotationSequence  RotationAngleUnits=deg  RotationStandardAxis=+Z  RotationAngle=0.0  RotationArbitraryAxis=[0 0 1]  FollAlignAxisA=+X  BaseAlignAxisA=+Y  FollAlignAxisB=+Y  BaseAlignAxisB=+Z  RotationSequenceAxes=BaseAxes  RotationSequence=XYZ  RotationSequenceAngles=[0, 0, 0]  RotationSequenceAnglesUnits=rad  RotationMatrix=[1 0 0; 0 1 0; 0 0 1]
  shoulder_pan_joint_AxisTransform : sm_lib/Frames and Transforms/Rigid Transform  TranslationMethod=Cartesian  TranslationStandardOffset=0  TranslationLengthUnit=m  TranslationStandardAxis=+Z  TranslationCartesianOffset=[0, 0, 0]  TranslationROffset=0  TranslationROffsetUnits=m  TranslationZOffset=0  TranslationZOffsetUnits=m  TranslationThetaOffset=0  TranslationThetaOffsetUnits=deg  RotationMethod=ArbitraryAxis  RotationAngleUnits=rad  RotationStandardAxis=+Z  RotationAngle=0  RotationArbitraryAxis=[1, 0, 0]  FollAlignAxisA=+X  BaseAlignAxisA=+Y  FollAlignAxisB=+Y  BaseAlignAxisB=+Z  RotationSequenceAxes=FollowerAxes  RotationSequence=XYX  RotationSequenceAngles=[0 0 0]  RotationSequenceAnglesUnits=deg  RotationMatrix=[1 0 0; 0 1 0; 0 0 1]
  shoulder_pan_joint_OriginTransform : sm_lib/Frames and Transforms/Rigid Transform  TranslationMethod=Cartesian  TranslationStandardOffset=0  TranslationLengthUnit=m  TranslationStandardAxis=+Z  TranslationCartesianOffset=[0, 0, 0.089159]  TranslationROffset=0  TranslationROffsetUnits=m  TranslationZOffset=0  TranslationZOffsetUnits=m  TranslationThetaOffset=0  TranslationThetaOffsetUnits=deg  RotationMethod=RotationSequence  RotationAngleUnits=deg  RotationStandardAxis=+Z  RotationAngle=0.0  RotationArbitraryAxis=[0 0 1]  FollAlignAxisA=+X  BaseAlignAxisA=+Y  FollAlignAxisB=+Y  BaseAlignAxisB=+Z  RotationSequenceAxes=BaseAxes  RotationSequence=XYZ  RotationSequenceAngles=[0, 0, 0]  RotationSequenceAnglesUnits=rad  RotationMatrix=[1 0 0; 0 1 0; 0 0 1]
  F : PMIOPort  Side=Left
  F2 : PMIOPort  Port=2  Side=Right
  connections:
  Inertia/RConn1 -- InertiaOriginTransform/RConn1
  ReferenceFrame/RConn1 -- InertiaOriginTransform/LConn1 -- shoulder_pan_joint_OriginTransform/LConn1 -- VisualOriginTransform/LConn1 -- F/RConn1
  Visual/RConn1 -- VisualOriginTransform/RConn1
  shoulder_pan_joint_AxisTransform/RConn1 -- F2/RConn1
  shoulder_pan_joint_AxisTransform/LConn1 -- shoulder_pan_joint_OriginTransform/RConn1
